simulink model "buck_converter"  (R2023a)
settings: Solver=VariableStepAuto  StartTime=0.0  StopTime=600e-3  RelTol=1e-3
libraries: spsSeriesRLCBranchLib x3, spsVoltageMeasurementLib x3, spsMosfetLib x2, spsCurrentMeasurementLib x1, spsDCVoltageSourceLib x1, sps_lib x1
settings Model: Creator=andre  LastModifiedBy=andre

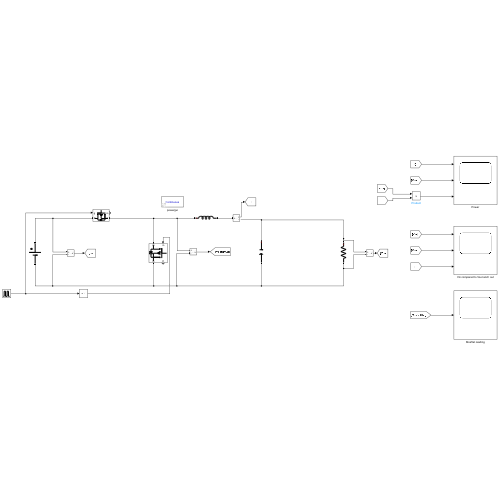
[thumbnail: Simulink's stored preview of the top-level diagram]
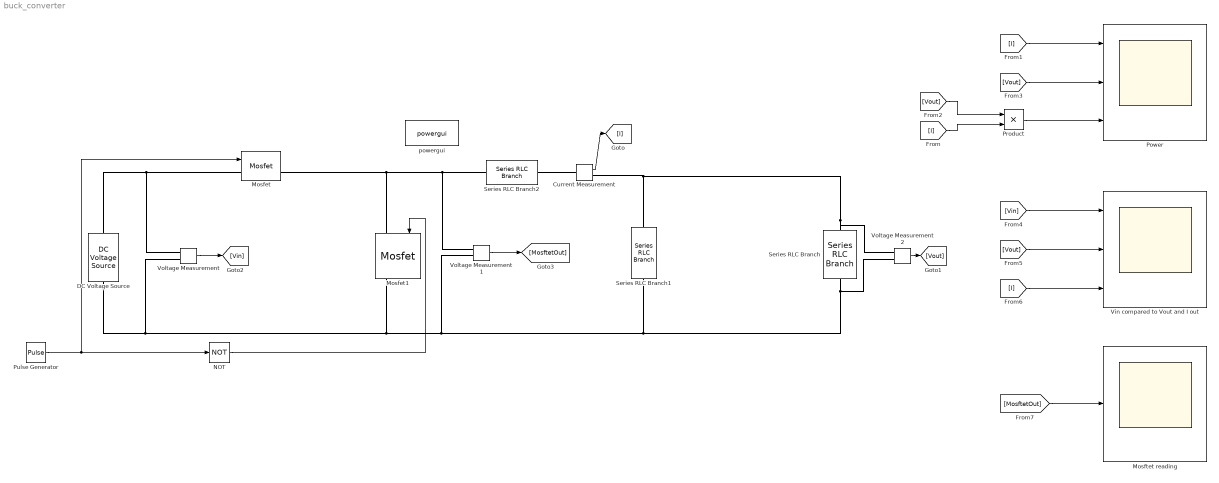
== system buck_converter ==
  Current Measurement : spsCurrentMeasurementLib/Current Measurement  PhasorSimulation=off  OutputType=Complex  PSBequivalent=0
  DC Voltage Source : spsDCVoltageSourceLib/DC Voltage Source  Amplitude=40  Measurements=None
  Mosfet : spsMosfetLib/Mosfet  Ron=0  Lon=0  Rd=0.0  Vfd=0  IC=0  Rs=inf  Cs=inf  Measurements=on
  Mosfet1 : spsMosfetLib/Mosfet  Ron=0  Lon=0  Rd=0  Vfd=0  IC=0  Rs=inf  Cs=inf  Measurements=on
  Mosftet reading : Scope
  NOT : Logic  Operator=NOT  AllPortsSameDT=off  OutDataTypeStr=boolean
  Power : Scope  NumInputPorts=3
  Product : Product
  Pulse Generator : DiscretePulseGenerator  PulseType=Time based  Period=1/27000  PulseWidth=70
  Series RLC Branch : spsSeriesRLCBranchLib/Series RLC Branch  LConnTagsString=__new0  RConnTagsString=__new0  BranchType=R  Resistance=1.96  Inductance=1e-3  SetiL0=off  InitialCurrent=0  Capacitance=1e-6  Setx0=off  InitialVoltage=0  Measurements=None
  Series RLC Branch1 : spsSeriesRLCBranchLib/Series RLC Branch  LConnTagsString=__new0  RConnTagsString=__new0  BranchType=C  Resistance=1  Inductance=1e-3  SetiL0=off  InitialCurrent=0  Capacitance=23.6e-6  Setx0=off  InitialVoltage=50  Measurements=None
  Series RLC Branch2 : spsSeriesRLCBranchLib/Series RLC Branch  LConnTagsString=__new0  RConnTagsString=__new0  BranchType=L  Resistance=1  Inductance=218e-6  SetiL0=off  InitialCurrent=0  Capacitance=1e-6  Setx0=off  InitialVoltage=0  Measurements=None
  Vin compared to Vout and I out : Scope  NumInputPorts=3
  Voltage Measurement : spsVoltageMeasurementLib/Voltage Measurement  PhasorSimulation=off  OutputType=Complex  PSBequivalent=0
  Voltage Measurement1 : spsVoltageMeasurementLib/Voltage Measurement  PhasorSimulation=off  OutputType=Complex  PSBequivalent=0
  Voltage Measurement2 : spsVoltageMeasurementLib/Voltage Measurement  PhasorSimulation=off  OutputType=Complex  PSBequivalent=0
  powergui : sps_lib/powergui  Priority=1  SimulationMode=Continuous  SampleTime=50e-6  frequency=60  Iterations=50  frequencyindice=0  Pbase=100e6  ErrMax=1e-4  UnitsV=kV  UnitsW=MW  buscounter=0  FunctionMessages=off  echomessages=off  EnableUseOfTLC=off  CurrentSourceSwitches=off  DisableSnubberDevices=off  DisableRonSwitches=off  DisableVfSwitches=off  DisplayEquations=off  AutomaticDiscreteSolvers=off  SolverType=Tustin/Backward Euler (TBE)  Interpol=off  ExternalGateDelay=off  methode=off  Ts=100  x0status=blocks  SPID=on  SwTol=0  HookPort=off  NonlinearTolerance=1e-4  nMaxIteration=100  ContinueOnMaxIteration=off  RestoreLinks=warning  ResistiveCurrentMeasurement=off  Frange=[0:2:500]  Ylog=off  Xlog=on  ShowGrid=off  save=off  variable=ZData  structure=0  ZoomFFT=off  StartTime=0.0  cycles=1  DisplayStyle=1  fundamental=60  FreqAxis=off  MaxFrequency=1000  frequencyindicesteady=1  RmsSteady=1  display=off
  wires:
  NOT/1 -> Mosfet1/1
  Pulse Generator/1 -> NOT/1, Mosfet/1
  Current Measurement/1 -> [I]
  [I] -> Product/2
  [I] -> Power/1
  Voltage Measurement2/1 -> [Vout]
  [Vout] -> Product/1
  [Vout] -> Power/2
  Product/1 -> Power/3
  Voltage Measurement/1 -> [Vin]
  [Vin] -> Vin compared to Vout and I out/1
  [Vout] -> Vin compared to Vout and I out/2
  [I] -> Vin compared to Vout and I out/3
  Voltage Measurement1/1 -> [MosftetOut]
  [MosftetOut] -> Mosftet reading/1
  connections:
  DC Voltage Source/LConn1 -- Voltage Measurement/LConn2 -- Voltage Measurement1/LConn2 -- Series RLC Branch1/RConn1 -- Voltage Measurement2/LConn2 -- Series RLC Branch/RConn1 -- Mosfet1/RConn1
  DC Voltage Source/RConn1 -- Voltage Measurement/LConn1 -- Mosfet/LConn1
  Series RLC Branch2/LConn1 -- Mosfet/RConn1 -- Mosfet1/LConn1 -- Voltage Measurement1/LConn1
  Series RLC Branch2/RConn1 -- Current Measurement/LConn1
  Series RLC Branch1/LConn1 -- Series RLC Branch/LConn1 -- Voltage Measurement2/LConn1 -- Current Measurement/RConn1
